simulink model "model_sterowania2015a"  (R2015a)
settings: Solver=ode45  StartTime=0.0  StopTime=sim_time  FixedStep=0.001  MaxStep=0.001  RelTol=1e-3
values from neighbouring files (symbols this model uses):
  a = 27.62    [parametry.m]
  b = -304.84    [parametry.m]
  c = 112.75    [parametry.m]
  d = -2.74    [parametry.m]
  g = 9.81    [parametry.m]
  m = 0.058    [parametry.m]
  R = 10    [linearize_model.m]    (also in parametry.m = 4.38)
  u_max = 12.28    [parametry.m]
libraries: simulink x1
settings Model: CovHtmlReporting=off  Creator=Student  LastModifiedBy=Student
settings DataIOCC: LimitDataPoints=off
settings GRTTargetCC: GeneratePreprocessorConditionals=Use local settings

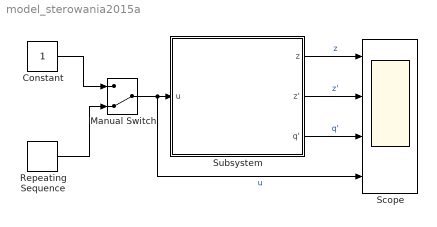
== system model_sterowania2015a ==
  Constant : Constant
  Manual Switch : ManualSwitch  CurrentSetting=0
  Repeating Sequence : simulink/Sources/Repeating Sequence  rep_seq_t=[0 1 10]  rep_seq_y=[0 1 1]
  Scope : Scope  NumInputPorts=4
      settings: ShowLegends=on  YMin=-0.00157~-2.02648~-0.34243~0.9  YMax=0.01417~0.33914~3.08191~1.1  SaveName=out
  Subsystem : Subsystem
  wires:
  Subsystem/3(q') -> Scope/3  "q'"
  Subsystem/2(z') -> Scope/2  "z'"
  Subsystem/1(z) -> Scope/1  "z"
  Repeating Sequence/1 -> Manual Switch/2
  Constant/1 -> Manual Switch/1
  Manual Switch/1 -> Scope/4, Subsystem/1(u)  "u"

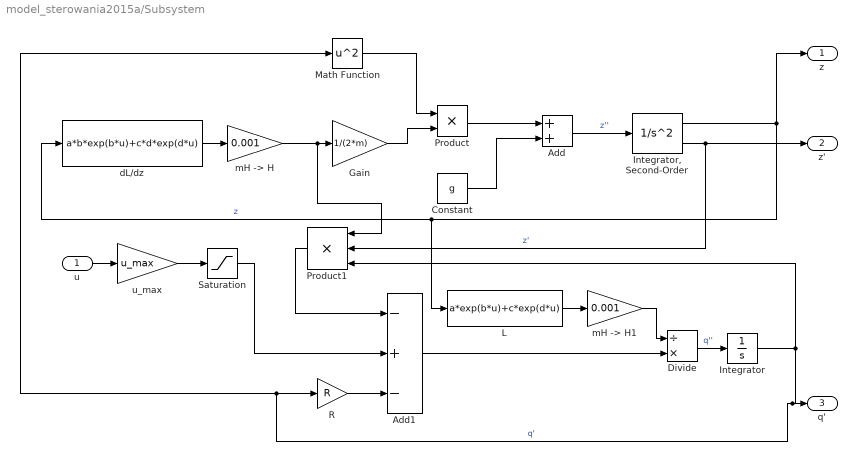
== system model_sterowania2015a/Subsystem ==
  u : Inport
  Add : Sum
  Add1 : Sum  Inputs=-+-
  Constant : Constant  Value=g
  Divide : Product  Inputs=/*
  Gain : Gain  Gain=1/(2*m)
  Integrator : Integrator
  "Integrator, Second-Order" : SecondOrderIntegrator  ICX=z0  LimitX=on  UpperLimitX=z0  LowerLimitX=0  ICDXDT=v0
  L : Fcn  Expr=a*exp(b*u)+c*exp(d*u)
  Math Function : Math  Operator=square  SaturateOnIntegerOverflow=on
  Product : Product
  Product1 : Product  Inputs=3
  R : Gain  Gain=R
  Saturation : Saturate  UpperLimit=12  LowerLimit=0
  dL/dz : Fcn  Expr=a*b*exp(b*u)+c*d*exp(d*u)
  "mH -> H" : Gain  Gain=0.001
  "mH -> H1" : Gain  Gain=0.001
  u_max : Gain  Gain=u_max
  z : Outport
  z' : Outport  Port=2
  q' : Outport  Port=3
  wires:
  Math Function/1 -> Product/1
  Constant/1 -> Add/2
  Product/1 -> Add/1
  Gain/1 -> Product/2
  "Integrator, Second-Order"/2 -> Product1/2, z'/1  "z'"
  R/1 -> Add1/3
  Add/1 -> "Integrator, Second-Order"/1  "z''"
  Saturation/1 -> Add1/2
  u/1 -> u_max/1
  u_max/1 -> Saturation/1
  Integrator/1 -> R/1, Math Function/1, q'/1, Product1/3  "q'"
  Divide/1 -> Integrator/1  "q''"
  "Integrator, Second-Order"/1 -> dL/dz/1, L/1, z/1  "z"
  Product1/1 -> Add1/1
  dL/dz/1 -> "mH -> H"/1
  Add1/1 -> Divide/2
  "mH -> H"/1 -> Product1/1, Gain/1
  L/1 -> "mH -> H1"/1
  "mH -> H1"/1 -> Divide/1
